simulink model "DTMF_Telefonie_Project_Crehul_Hornai"  (R2018b)
settings: Solver=VariableStepAuto  StartTime=0.0  StopTime=100  RelTol=1e-3
undefined symbols (not defined in the file): fdesignblkfcn, gcbh
libraries: simulink x12, dspfdesign x7
(part 4 of 4)

== system DTMF_Telefonie_Project_Crehul_Hornai/DTMF Detector and Decoder/Subsystem1/941Hz Bandpass Filter ==
  In : Inport
  Generated Filter Block : DiscreteFir  Tag=BlockMethodSubSystem  Coefficients=[-8.44056331013192832e-05 -0.00120076765466288395 -4.49460330017917694e-05 -5.80375074727710672e-05 3.71220945475457108e-05 0.000118681403074774063 0.000163532285663090952 0.000153192658350644203 8.81802496868124849e-05 -1.15090324239146489e-05 -0.000112520435481172214 -0.000179188261857551802 -0.000186197823069253411 -0.000128040314610888801 -2.19992603277147554e-05 9.68589974523585017e-05 0.000187220804360153692 0.000215990628509714214 0.000170217378145278342 6.2780285369345469e-05 -7.12325046840682979e-05 -0.000185802715721613507 -0.000239941578438043637 -0.000212215712394431938 -0.000109213954392370051 3.58011767851456773e-05 0.000173569581659991593 0.000255620241680421846 0.000251309357120219751 0.000159254217179292864 8.72829926178339759e-06 -0.000149597686606933619 -0.000260741507796367878 -0.000284529126023186406 -0.000210116880178106335 -6.0656051708186869e-05 0.000113905606048071944 0.000253489348119548675 0.000308644487204928753 0.000258079260682311112 0.000116857172512214918 -6.80195720963314225e-05 -0.000233249289015476931 -0.000320994113519973542 -0.000299201291805407661 -0.000173389665408685674 1.46316441594936741e-05 0.000200664985482552986 0.000320229566575600834 0.000330992811689179037 0.000227820406739258292 4.49579610132861714e-05 -0.000155401665291071282 -0.000304381185989563104 -0.0003500785241561842 -0.000275698609958245318 -0.000105649666291156963 0.000102003720656118499 0.000275629109764951197 0.000354716369189133458 0.000312084739020725491 0.000162815486417645873 -4.17100420797603022e-05 -0.000232567410926342146 -0.000343758426667818912 -0.000335632361658280676 -0.000212693152095347077 -1.98258717727487541e-05 0.000180837929206370312 0.000315633444353022861 0.000342426974179392703 0.000251722824589998347 7.66630020283598013e-05 -0.000121384545587020795 -0.000274664055250637112 -0.000331271251999935737 -0.000274325204948291804 -0.000125578863763076034 6.15561973850011846e-05 0.000222456027468240545 0.000302856498734454941 0.00027823975906371705 0.000160535944450468035 -6.38352457606536824e-06 -0.000163914844384561786 -0.000258739683562109657 -0.000261894809525833286 -0.000176957416038562291 -3.79350047082052021e-05 0.000104860307597674879 0.00020258352024135425 0.000225437206503371819 0.000171333860800437814 6.51924684081792909e-05 -5.23519403415369103e-05 -0.000140077966052497852 -0.000171385645770063969 -0.000142085490950829896 -7.01631940463882774e-05 1.3555484126797553e-05 7.7895664761008676e-05 0.000103567927089865102 8.88378943873165713e-05 4.82498000258914188e-05 4.03976979663097768e-06 -2.42009024468171501e-05 -2.84156444051702175e-05 -1.42895329436349765e-05 2.54694488264332416e-06 5.87092531655520206e-06 -1.22404141900698198e-05 -4.5754836074443872e-05 -7.66543022211142115e-05 -8.26555404750162643e-05 -4.89852058675235079e-05 2.24363061895297379e-05 0.000109616309768043602 0.000177140658288773455 0.000189576612364088069 0.000128119526094988914 1.51210694736559932e-06 -0.00015227757973797901 -0.000277110922767717931 -0.000318136040806503255 -0.000244648460785109158 -6.6615962030855069e-05 0.000163375545795660512 0.000365539498093927768 0.000459783886642139495 0.000395862378137934727 0.000177477363732662284 -0.000132325890835236257 -0.000429856844465511623 -0.000603877589419131834 -0.000575949892525186215 -0.00033609444631688861 5.05942811122226353e-05 0.000456822932025119854 0.00073670351806165641 0.000776696913351912011 0.000540239235490173994 8.87284162172630831e-05 -0.000433500650005991814 -0.000843632230759632624 -0.000984962414002010442 -0.000784816677329444189 -0.000288546730118970421 0.0003486416663457884 0.000908739543324476652 0.00118577347007898203 0.00106013159880728454 0.000548564284696077126 -0.000193158925505173174 -0.000915990068260141128 -0.00136139584583722345 -0.00135261229498154505 -0.000863884959136611589 -3.85929128784020812e-05 0.000850875180967379172 0.00149296361096120365 0.00164512254368231461 0.00122485688623547874 0.00034789073217438547 -0.000701185957402331353 ...(+11784 chars)]  InputProcessing=Columns as channels (frame based)
  Out : Outport
  wires:
  In/1 -> Generated Filter Block/1
  Generated Filter Block/1 -> Out/1
